simulink library "groundStationMSD_ul"  (R2018b)
settings: Solver=VariableStepAuto  StartTime=0.0  StopTime=10.0  RelTol=1e-3
settings Model: Creator=mcobb  LastModifiedBy=mcobb

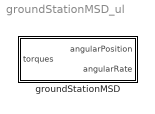
== system groundStationMSD_ul ==
  groundStationMSD : Subsystem  mask{J=1, b=1, k=1, theta_0=0, omega_0=0}
      mask prompts: J "Rotational Inertia"; b "Damping Coefficient"; k "Spring Constant"; theta_0 "Initial Position [rad]"; omega_0 "Initial Velocity [rad/s]"
      mask DialogControl Container3 Prompt: Initial Conditions

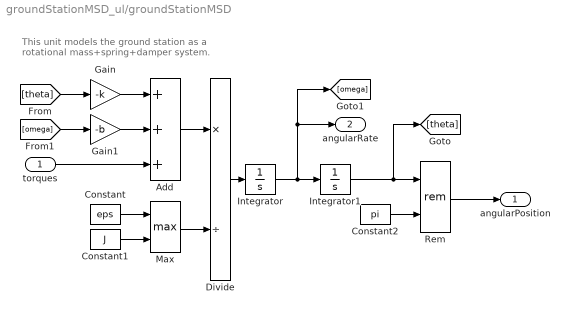
== system groundStationMSD_ul/groundStationMSD ==
  note: This unit models the ground station as
      | a rotational mass+spring+damper system.
  torques : Inport
  Add : Sum  Inputs=+++
  Constant : Constant  Value=eps
  Constant1 : Constant  Value=J
  Constant2 : Constant  Value=pi
  Divide : Product  Inputs=*/
  Gain : Gain  Gain=-k
  Gain1 : Gain  Gain=-b
  Integrator : Integrator  InitialCondition=omega_0
  Integrator1 : Integrator  InitialCondition=theta_0
  Max : MinMax  Function=max  Inputs=2
  Rem : Math  Operator=rem  SaturateOnIntegerOverflow=on
  angularPosition : Outport
  angularRate : Outport  Port=2
  wires:
  Max/1 -> Divide/2
  Constant/1 -> Max/1
  Divide/1 -> Integrator/1
  Constant1/1 -> Max/2
  [theta] -> Gain/1
  Gain/1 -> Add/1
  [omega] -> Gain1/1
  Gain1/1 -> Add/2
  torques/1 -> Add/3
  Add/1 -> Divide/1
  Integrator/1 -> angularRate/1, [omega], Integrator1/1
  Integrator1/1 -> [theta], Rem/1
  Rem/1 -> angularPosition/1
  Constant2/1 -> Rem/2
